simulink model "mysim"  (R2021b)
settings: Solver=ode45  StartTime=0.0  StopTime=t_stop  MaxStep=1e-4  MinStep=1e-5  RelTol=1e-3
libraries: cstblocks x2
settings Model: Creator=phos  LastModifiedBy=phos
settings SolverCC: InitialStep=1e-5

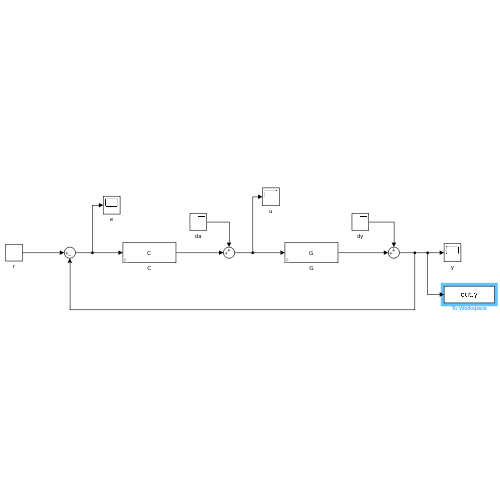
[thumbnail: Simulink's stored preview of the top-level diagram]
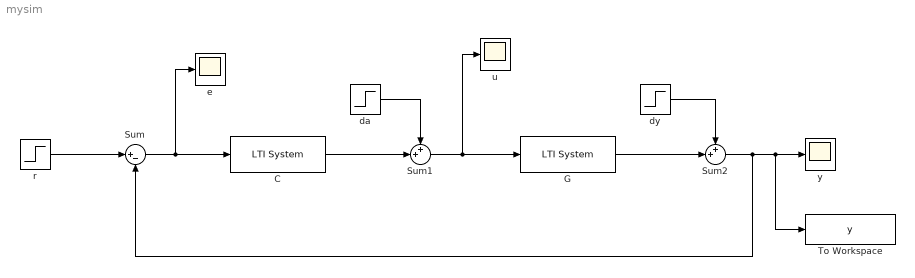
== system mysim ==
  C : cstblocks/LTI System  sys=C  IC=[]
  G : cstblocks/LTI System  sys=G  IC=[]
  Sum : Sum  Inputs=|+-
  Sum1 : Sum  Inputs=++|
  Sum2 : Sum  Inputs=++|
  To Workspace : ToWorkspace  VariableName=y  SaveFormat=Timeseries  SampleTime=-1
  da : Step  Time=0  After=0  SampleTime=0
  dy : Step  Time=0  After=0  SampleTime=0
  e : Scope
  r : Step  Time=0  SampleTime=0
  u : Scope
  y : Scope
  wires:
  Sum/1 -> e/1, C/1
  C/1 -> Sum1/2
  Sum1/1 -> u/1, G/1
  G/1 -> Sum2/2
  r/1 -> Sum/1
  dy/1 -> Sum2/1
  Sum2/1 -> To Workspace/1, y/1, Sum/2
  da/1 -> Sum1/1
